simulink model "attitude_dynamics"  (R2022a)
settings: Solver=VariableStepAuto  StartTime=0.0  StopTime=1000  RelTol=1e-3
libraries: shared6dof x1, aerolibanim x1, sharedtransform x1
settings Model: Creator=samuel  LastModifiedBy=samuel

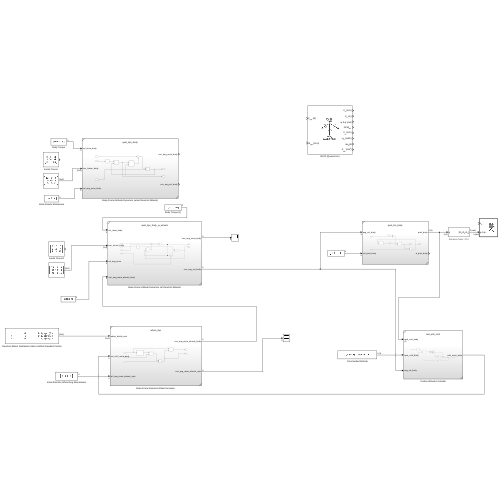
[thumbnail: Simulink's stored preview of the top-level diagram]
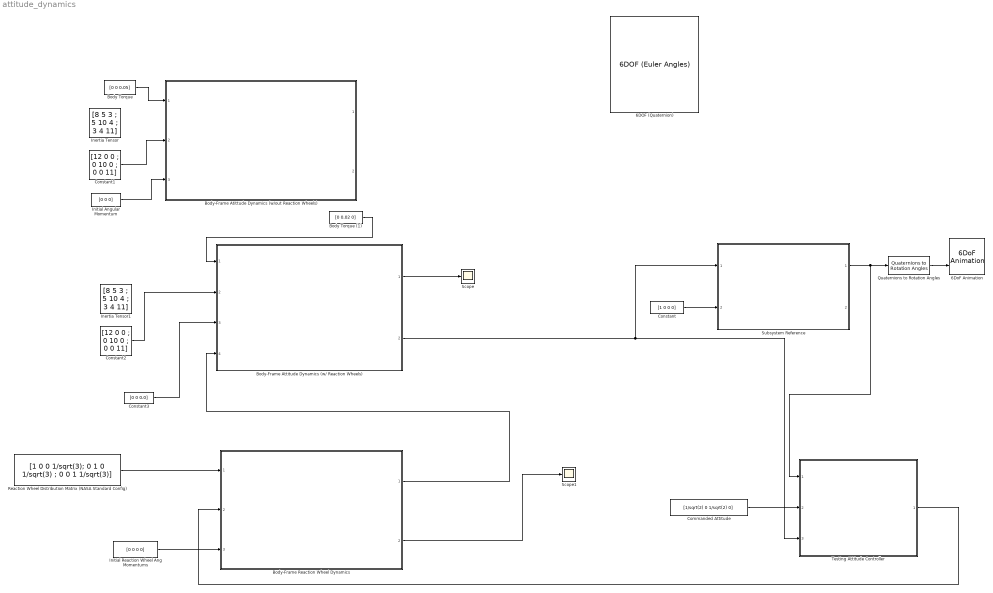
== system attitude_dynamics ==
  6DOF (Quaternion) : shared6dof/6DOF (Euler Angles)  units=Metric (MKS)  mtype=Fixed  rep=Quaternion  xme_0=[0 0 0]  Vm_0=[0 0 0]  eul_0=[0 0 0]  pm_0=[0 0 0]  mass_0=1.0  mass_e=0.5  mass_f=2.0  inertia=eye(3)  inertia_e=eye(3)  inertia_f=2*eye(3)  k_quat=1.0  vre_flag=on  abi_flag=off  aMode=0  xme_statename=''  Vm_statename=''  eul_statename=''  quat_statename=''  pm_statename=''  mass_statename=''
      settings: SourceProductBaseCode=AE,PW,DR,MT,VE
  6DoF Animation : aerolibanim/6DoF Animation  u1=[0 4000 -2000 2000 -5000 -3000]  u2=0.1  u3=1.0  u4=[4000 0 -5000]  u5=Fixed position  u6=[5 5 5]  u7=10  u8=on
  Body Torque : Constant  Value=[0 0 0.05]
  Body Torque (1) : Constant  Value=[0 0.02 0]
  Body-Frame Atittude Dynamics (w/out Reaction Wheels) : Subsystem  ReferencedSubsystem=quat_dyn_body
  Body-Frame Attitude Dynamics (w/ Reaction Wheels) : Subsystem  ReferencedSubsystem=quat_dyn_body_w_wheels
  Body-Frame Reaction Wheel Dynamics : Subsystem  ReferencedSubsystem=wheel_dyn
  Commanded Attitude : Constant  Value=[1/sqrt(2) 0 1/sqrt(2) 0]
  Constant : Constant  Value=[1 0 0 0]
  Constant1 : Constant  Value=[12 0 0 ; 0 10 0 ; 0 0 11]
  Constant2 : Constant  Value=[12 0 0 ; 0 10 0 ; 0 0 11]
  Constant3 : Constant  Value=[0 0 0.0]
  Inertia Tensor : Constant  Value=[8 5 3 ; 5 10 4 ; 3 4 11]
  Inertia Tensor1 : Constant  Value=[8 5 3 ; 5 10 4 ; 3 4 11]
  Initial Angular Momentum : Constant  Value=[0 0 0]
  Initial Reaction Wheel Ang Momentums : Constant  Value=[0 0 0 0]
  Quaternions to Rotation Angles : sharedtransform/Quaternions to Rotation Angles  rotationOrder=ZYX  aMode=aMode
      settings: SourceProductBaseCode=AE,PW,DR,MT,VE
  Reaction Wheel Distribution Matrix (NASA Standard Config) : Constant  Value=[1 0 0 1/sqrt(3); 0 1 0 1/sqrt(3) ; 0 0 1 1/sqrt(3)]
  Scope : Scope
  Scope1 : Scope
  Subsystem Reference : Subsystem  ReferencedSubsystem=quat_kin_body
  Testing Attitude Controller : Subsystem  ReferencedSubsystem=test_attit_cntrl
  wires:
  Quaternions to Rotation Angles/1 -> 6DoF Animation/2
  Constant/1 -> Subsystem Reference/2
  Subsystem Reference/1 -> Testing Attitude Controller/1, Quaternions to Rotation Angles/1
  Body Torque/1 -> Body-Frame Atittude Dynamics (w/out Reaction Wheels)/1
  Constant1/1 -> Body-Frame Atittude Dynamics (w/out Reaction Wheels)/2
  Initial Angular Momentum/1 -> Body-Frame Atittude Dynamics (w/out Reaction Wheels)/3
  Body-Frame Attitude Dynamics (w/ Reaction Wheels)/2 -> Testing Attitude Controller/3, Subsystem Reference/1
  Body Torque (1)/1 -> Body-Frame Attitude Dynamics (w/ Reaction Wheels)/1
  Constant2/1 -> Body-Frame Attitude Dynamics (w/ Reaction Wheels)/2
  Constant3/1 -> Body-Frame Attitude Dynamics (w/ Reaction Wheels)/3
  Body-Frame Attitude Dynamics (w/ Reaction Wheels)/1 -> Scope/1
  Reaction Wheel Distribution Matrix (NASA Standard Config)/1 -> Body-Frame Reaction Wheel Dynamics/1
  Initial Reaction Wheel Ang Momentums/1 -> Body-Frame Reaction Wheel Dynamics/3
  Body-Frame Reaction Wheel Dynamics/1 -> Body-Frame Attitude Dynamics (w/ Reaction Wheels)/4
  Body-Frame Reaction Wheel Dynamics/2 -> Scope1/1
  Commanded Attitude/1 -> Testing Attitude Controller/2
  Testing Attitude Controller/1 -> Body-Frame Reaction Wheel Dynamics/2
